simulink model "legoSS_MCC_sim"  (R2025a)
settings: Solver=ode45  StartTime=0.0  StopTime=50  RelTol=1e-3  EnableMultiTasking=on
values from neighbouring files (symbols this model uses):
  A = [0 1;-denom(3) -denom(2)]    [AncienTest.m]    (also in Test.m)
  B = [num(2) num(3)]'    [AncienTest.m]    (also in Test.m)
  K_corr = acker(Ad,Bd,poles_souhaites)    [AncienTest.m]    (also in Test.m)
  S_corr = inv(Cd*inv(eye(2)-Ad+Bd*K_corr)*Bd)    [AncienTest.m]    (also in Test.m)
  Te = 1/100    (= 0.01)    [AncienTest.m]    (also in Test.m)
settings Model: Creator=jacques  LastModifiedBy=carol
settings SolverCC: AlgebraicLoopSolver=TrustRegion
settings DataIOCC: LimitDataPoints=on  SaveFormat=Array  SignalLoggingSaveFormat=ModelDataLogs  ReturnWorkspaceOutputs=off
settings OptimizationCC: ExpressionDepthLimit=2147483647.0  LifeSpan=inf
settings DebuggingCC: UnderspecifiedInitializationDetection=Classic  MergeDetectMultiDrivingBlocksExec=none  SolverPrmCheckMsg=warning  FcnCallInpInsideContextMsg=warning  UnconnectedInputMsg=warning  UnconnectedOutputMsg=warning  UnconnectedLineMsg=warning  StateNameClashWarn=warning  SFUnexpectedBacktrackingDiag=warning  SFNoUnconditionalDefaultTransitionDiag=warning  SFExecutionAtInitializationDiag=none  ArithmeticOperatorsInVariantConditions=warning
settings HardwareCC: ProdBitPerPointer=32.0  ProdBitPerSizeT=32.0  ProdBitPerPtrDiffT=32.0  ProdLargestAtomicFloat=None  ProdIntDivRoundTo=Undefined  ProdEndianess=Unspecified  ProdWordSize=32.0  ProdHWDeviceType=32-bit Generic
settings ModelReferenceCC: EnableRefExpFcnMdlSchedulingChecks=on  PropagateSignalLabelsOutOfModel=off
settings SFSimCC: SimUseLocalCustomCode=off  CustomCodeUndefinedFunction=UseInterfaceOnly
settings RTWCC: RTWUseLocalCustomCode=off  GPUComputeCapability=3.5  DLArmComputeVersion=19.05
settings CodeAppCC: StateflowObjectComments=on
settings GRTTargetCC: TargetLangStandard=C89/C90 (ANSI)  CombineOutputUpdateFcns=off  GRTInterface=on
settings ConfigComp: CovMetricSettings=dw  CovSaveCumulativeToWorkspaceVar=on  CovSaveSingleToWorkspaceVar=on  CovExternalEMLEnable=off

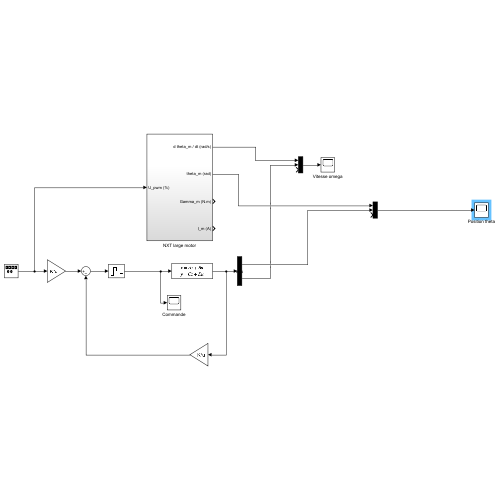
[thumbnail: Simulink's stored preview of the top-level diagram]
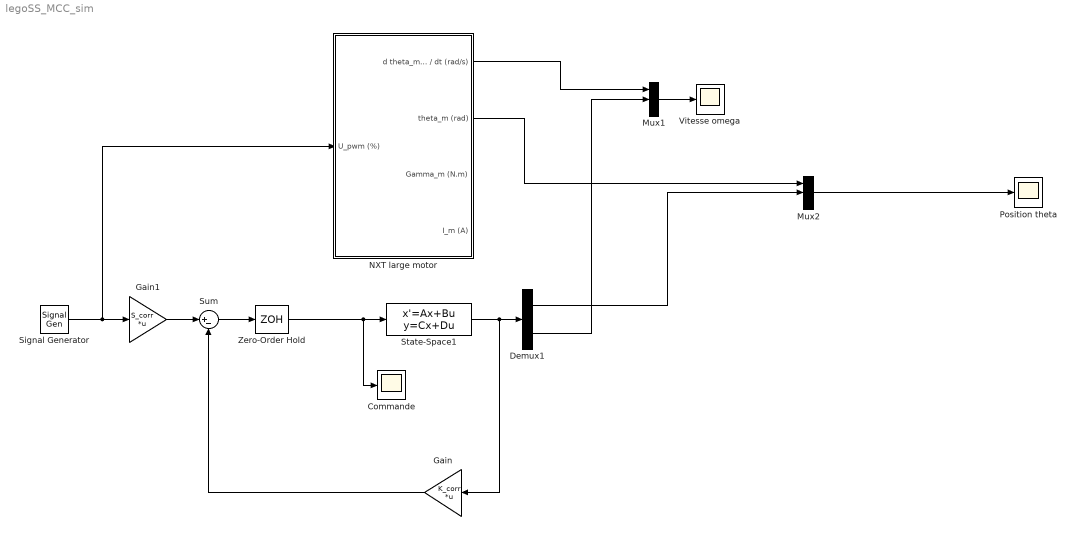
== system legoSS_MCC_sim ==
  Commande : Scope
      settings: ActiveDisplayYMinimum=-3.3187989202520205  ActiveDisplayYMaximum=3.3187989202430117  DataLoggingMaxPoints=5000000  DataLoggingVariableName=ScopeData2
  Demux1 : Demux  Outputs=2
      settings: DisplayOption=none
  Gain : Gain  Gain=K_corr  Multiplication=Matrix(K*u)
  Gain1 : Gain  Gain=S_corr  Multiplication=Matrix(K*u)
  Mux1 : Mux  Inputs=3
  Mux2 : Mux  Inputs=3
  NXT large motor : Subsystem
  Position theta : Scope
      settings: ActiveDisplayYMinimum=-1.5007470192815222  ActiveDisplayYMaximum=1.5007470192645822  DataLoggingMaxPoints=5000000
  Signal Generator : SignalGenerator  WaveForm=square  Frequency=0.1
  State-Space1 : StateSpace  A=A  B=B  C=eye(2)  D=[0;0]  InitialCondition=0
  Sum : Sum  Inputs=|+-
  Vitesse omega : Scope
      settings: ActiveDisplayYMinimum=-0.23924134896009266  ActiveDisplayYMaximum=0.36318158115297844  DataLoggingMaxPoints=5000000
  Zero-Order Hold : ZeroOrderHold  SampleTime=Te
  wires:
  Signal Generator/1 -> Gain1/1, NXT large motor/1(U_pwm (%))
  State-Space1/1 -> Gain/1, Demux1/1
  Mux1/1 -> Vitesse omega/1
  NXT large motor/2(theta_m (rad)) -> Mux2/1
  Mux2/1 -> Position theta/1
  NXT large motor/1(d theta_m / dt (rad/s)) -> Mux1/1
  Sum/1 -> Zero-Order Hold/1
  Zero-Order Hold/1 -> Commande/1, State-Space1/1
  Gain/1 -> Sum/2
  Demux1/1 -> Mux2/2
  Demux1/2 -> Mux1/2
  Gain1/1 -> Sum/1

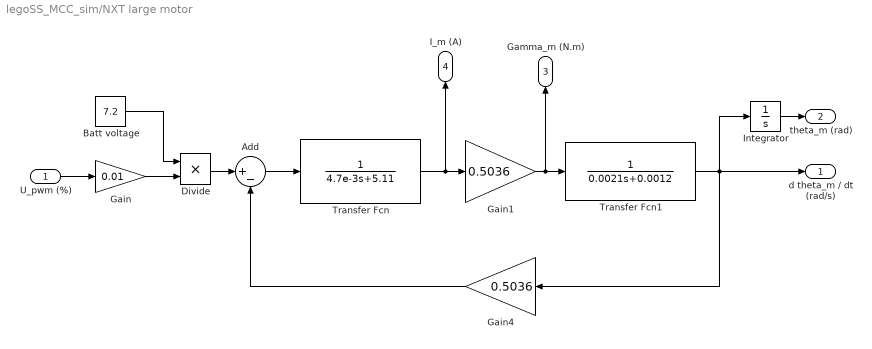
== system legoSS_MCC_sim/NXT large motor ==
  U_pwm (%) : Inport
  Add : Sum  Inputs=|+-
  Batt voltage : Constant  Value=7.2
  Divide : Product  Inputs=**
  Gain : Gain  Gain=0.01
  Gain1 : Gain  Gain=0.5036
  Gain4 : Gain  Gain=0.5036
  Integrator : Integrator
  Transfer Fcn : TransferFcn  Denominator=[4.7e-3 5.11]
  Transfer Fcn1 : TransferFcn  Denominator=[0.0021 0.0012]
  d theta_m / dt (rad/s) : Outport
  theta_m (rad) : Outport  Port=2
  Gamma_m (N.m) : Outport  Port=3
  I_m (A) : Outport  Port=4
  wires:
  Batt voltage/1 -> Divide/1
  Gain/1 -> Divide/2
  Divide/1 -> Add/1
  Add/1 -> Transfer Fcn/1
  Transfer Fcn/1 -> Gain1/1, I_m (A)/1
  Gain1/1 -> Transfer Fcn1/1, Gamma_m (N.m)/1
  Transfer Fcn1/1 -> Integrator/1, Gain4/1, d theta_m / dt (rad/s)/1
  Gain4/1 -> Add/2
  U_pwm (%)/1 -> Gain/1
  Integrator/1 -> theta_m (rad)/1
